simulink model "Quadcopter_Auto_Hinf_Discrete"  (R2016b)
settings: Solver=ode45  StartTime=0.0  StopTime=100  RelTol=1e-3  EnableMultiTasking=on
undefined symbols (not defined in the file): A, B, C, DiscIntNeverNeededParam, g, K_lqi, m, sigbuilder_block, Ts, X0
libraries: simulink x1
settings Model: Creator=Toshiba  LastModifiedBy=AAstudillo
settings DataIOCC: LimitDataPoints=on  SaveFormat=Array  SignalLoggingSaveFormat=ModelDataLogs
settings OptimizationCC: LifeSpan=inf
settings DebuggingCC: SolverPrmCheckMsg=warning  MultiTaskDSMMsg=warning  MultiTaskCondExecSysMsg=none  SFUnexpectedBacktrackingDiag=warning  SFNoUnconditionalDefaultTransitionDiag=warning  SFExecutionAtInitializationDiag=none
settings HardwareCC: ProdBitPerPointer=32  ProdBitPerSizeT=32  ProdBitPerPtrDiffT=32  ProdLargestAtomicFloat=None  ProdIntDivRoundTo=Undefined  ProdEndianess=Unspecified  ProdWordSize=32  ProdHWDeviceType=32-bit Generic
settings ModelReferenceCC: PropagateSignalLabelsOutOfModel=off
settings GRTTargetCC: TargetLangStandard=C89/C90 (ANSI)  GeneratePreprocessorConditionals=Disable all
settings ConfigComp: CovMetricSettings=dw  CovHtmlReporting=on  CovSaveCumulativeToWorkspaceVar=on  CovSaveSingleToWorkspaceVar=on  CovExternalEMLEnable=off

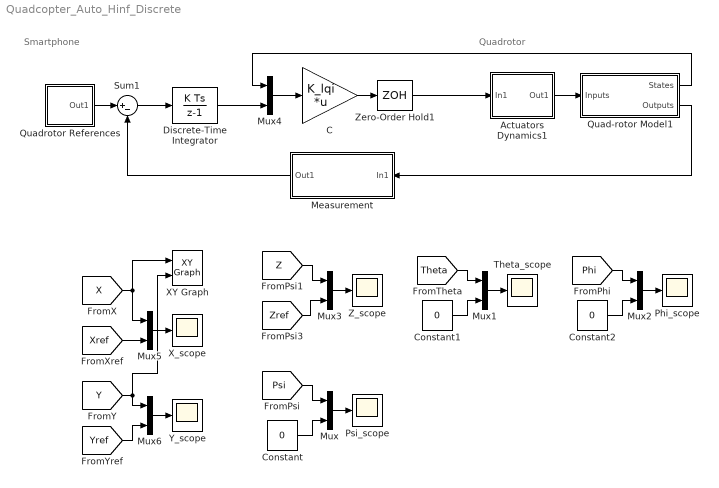
== system Quadcopter_Auto_Hinf_Discrete ==
  note: Quadrotor
  note: Smartphone
  Actuators Dynamics1 : Subsystem
  C : Gain  Gain=K_lqi  Multiplication=Matrix(K*u)
  Constant : Constant  Value=0
  Constant1 : Constant  Value=0
  Constant2 : Constant  Value=0
  Discrete-Time Integrator : DiscreteIntegrator  InitialConditionSetting=State (most efficient)  SampleTime=Ts  UpperSaturationLimit=10  LowerSaturationLimit=-10  ICPrevOutput=DiscIntNeverNeededParam  ICPrevScaledInput=DiscIntNeverNeededParam
  Measurement : Subsystem
  Mux{,1..6} (7 alike) : Mux  Inputs=2
  Phi_scope : Scope
  Psi_scope : Scope
  Quad-rotor Model1 : Subsystem
  Quadrotor References : Subsystem
  Sum1 : Sum  Inputs=|+-
  Theta_scope : Scope
  XY Graph : simulink/Sinks/XY Graph  xmin=-1  xmax=3  ymin=-1  ymax=3  st=Ts
  X_scope : Scope
  Y_scope : Scope
  Z_scope : Scope
  Zero-Order Hold1 : ZeroOrderHold  SampleTime=Ts
  wires:
  Mux/1 -> Psi_scope/1
  Mux1/1 -> Theta_scope/1
  Mux2/1 -> Phi_scope/1
  [Psi] -> Mux/1
  Constant/1 -> Mux/2
  [Theta] -> Mux1/1
  [Phi] -> Mux2/1
  Constant2/1 -> Mux2/2
  Mux3/1 -> Z_scope/1
  [Z] -> Mux3/1
  C/1 -> Zero-Order Hold1/1
  Quad-rotor Model1/1(States) -> Mux4/1
  Mux4/1 -> C/1
  Quadrotor References/1(Out1) -> Sum1/1
  Sum1/1 -> Discrete-Time Integrator/1
  Discrete-Time Integrator/1 -> Mux4/2
  Measurement/1(Out1) -> Sum1/2
  Quad-rotor Model1/2(Outputs) -> Measurement/1(In1)
  Zero-Order Hold1/1 -> Actuators Dynamics1/1(In1)
  Actuators Dynamics1/1(Out1) -> Quad-rotor Model1/1(Inputs)
  Constant1/1 -> Mux1/2
  [Zref] -> Mux3/2
  Mux5/1 -> X_scope/1
  Mux6/1 -> Y_scope/1
  [X] -> XY Graph/1, Mux5/1
  [Xref] -> Mux5/2
  [Y] -> Mux6/1, XY Graph/2
  [Yref] -> Mux6/2

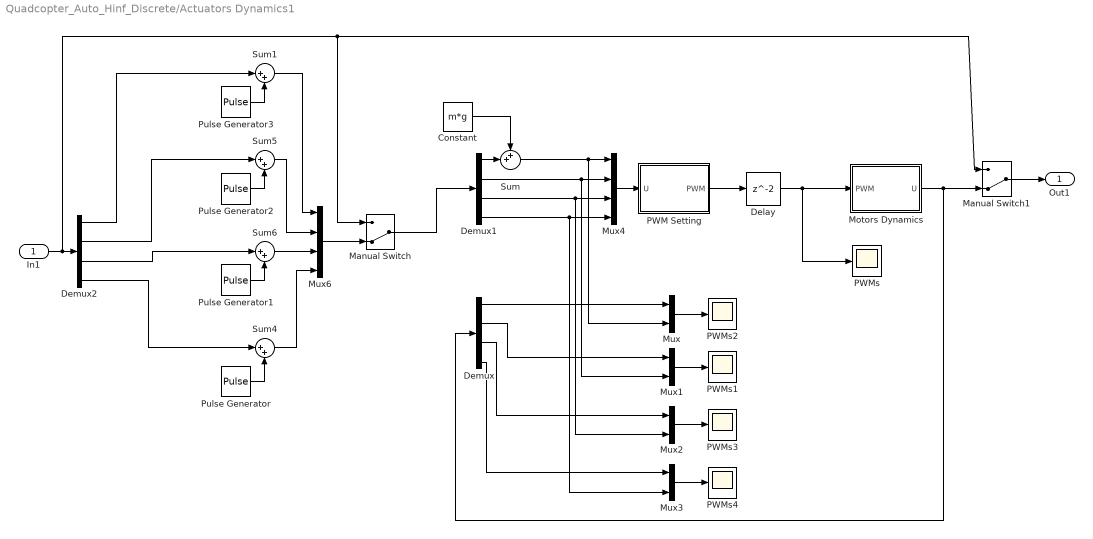
== system Quadcopter_Auto_Hinf_Discrete/Actuators Dynamics1 ==
  In1 : Inport
  Constant : Constant  Value=m*g  VectorParams1D=off  SampleTime=Ts
  Delay : Delay  SampleTime=Ts/10
  Demux : Demux
  Demux1 : Demux
  Demux2 : Demux
  Manual Switch : ManualSwitch  CurrentSetting=0
  Manual Switch1 : ManualSwitch  CurrentSetting=0
  Motors Dynamics : MATLAB Function  TreatAsAtomicUnit=on
  Mux{,1..3} (4 alike) : Mux  Inputs=2
  Mux4 : Mux
  Mux6 : Mux
  PWM Setting : MATLAB Function  TreatAsAtomicUnit=on
  PWMs{,1..4} (5 alike) : Scope
  Pulse Generator : DiscretePulseGenerator  PulseType=Time based  Amplitude=0.05  Period=20  PulseWidth=10  PhaseDelay=10
  Pulse Generator1 : DiscretePulseGenerator  PulseType=Time based  Amplitude=0.1  Period=15  PulseWidth=10  PhaseDelay=5
  Pulse Generator2 : DiscretePulseGenerator  PulseType=Time based  Amplitude=0.2  Period=17  PhaseDelay=15
  Pulse Generator3 : DiscretePulseGenerator  PulseType=Time based  Amplitude=0.1  Period=15  PhaseDelay=15
  Sum : Sum  Inputs=++|
  Sum{1,4..6} (4 alike) : Sum  Inputs=|++
  Out1 : Outport
  wires:
  Motors Dynamics/1(U) -> Manual Switch1/2, Demux/1
  Mux/1 -> PWMs2/1
  Mux1/1 -> PWMs1/1
  Mux2/1 -> PWMs3/1
  Mux3/1 -> PWMs4/1
  Demux/1 -> Mux/1
  Demux/2 -> Mux1/1
  Demux/3 -> Mux2/1
  Demux/4 -> Mux3/1
  Constant/1 -> Sum/1
  Demux1/1 -> Sum/2
  Sum/1 -> Mux/2, Mux4/1
  Demux1/2 -> Mux1/2, Mux4/2
  Demux1/3 -> Mux2/2, Mux4/3
  Demux1/4 -> Mux3/2, Mux4/4
  Mux4/1 -> PWM Setting/1(U)
  PWM Setting/1(PWM) -> Delay/1
  Delay/1 -> PWMs/1, Motors Dynamics/1(PWM)
  Pulse Generator/1 -> Sum4/2
  Pulse Generator1/1 -> Sum6/2
  Pulse Generator2/1 -> Sum5/2
  In1/1 -> Manual Switch1/1, Manual Switch/1, Demux2/1
  Demux2/2 -> Sum5/1
  Demux2/3 -> Sum6/1
  Demux2/4 -> Sum4/1
  Sum5/1 -> Mux6/2
  Sum6/1 -> Mux6/3
  Sum4/1 -> Mux6/4
  Pulse Generator3/1 -> Sum1/2
  Demux2/1 -> Sum1/1
  Sum1/1 -> Mux6/1
  Manual Switch/1 -> Demux1/1
  Mux6/1 -> Manual Switch/2
  Manual Switch1/1 -> Out1/1

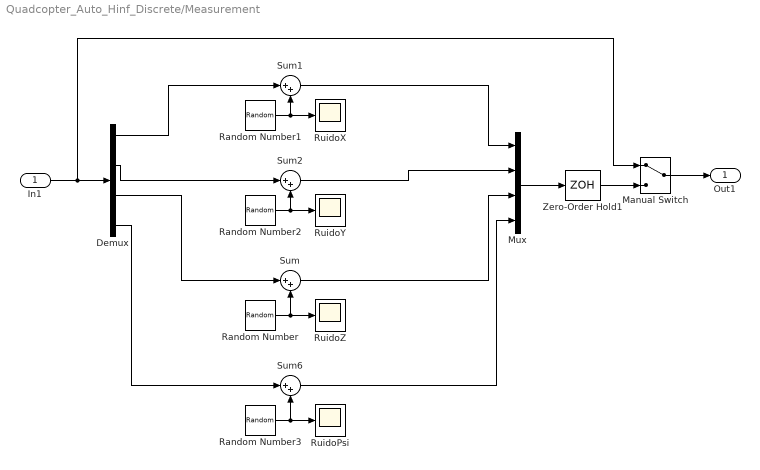
== system Quadcopter_Auto_Hinf_Discrete/Measurement ==
  In1 : Inport
  Demux : Demux
  Manual Switch : ManualSwitch
  Mux : Mux
  Random Number : RandomNumber  Variance=0.005  SampleTime=Ts*100
  Random Number1 : RandomNumber  Variance=0.05  SampleTime=Ts*100
  Random Number2 : RandomNumber  Variance=0.05  SampleTime=Ts*100
  Random Number3 : RandomNumber  Variance=0.00125  SampleTime=Ts
  RuidoPsi : Scope
  RuidoX : Scope
  RuidoY : Scope
  RuidoZ : Scope
  Sum{,1..2,6} (4 alike) : Sum  Inputs=|++
  Zero-Order Hold1 : ZeroOrderHold  SampleTime=Ts
  Out1 : Outport
  wires:
  Mux/1 -> Zero-Order Hold1/1
  Random Number/1 -> Sum/2, RuidoZ/1
  Demux/3 -> Sum/1
  Demux/1 -> Sum1/1
  Random Number2/1 -> RuidoY/1, Sum2/2
  Demux/2 -> Sum2/1
  Random Number1/1 -> RuidoX/1, Sum1/2
  Sum1/1 -> Mux/1
  Sum2/1 -> Mux/2
  Sum/1 -> Mux/3
  Random Number3/1 -> Sum6/2, RuidoPsi/1
  Demux/4 -> Sum6/1
  Sum6/1 -> Mux/4
  Manual Switch/1 -> Out1/1
  Zero-Order Hold1/1 -> Manual Switch/2
  In1/1 -> Manual Switch/1, Demux/1

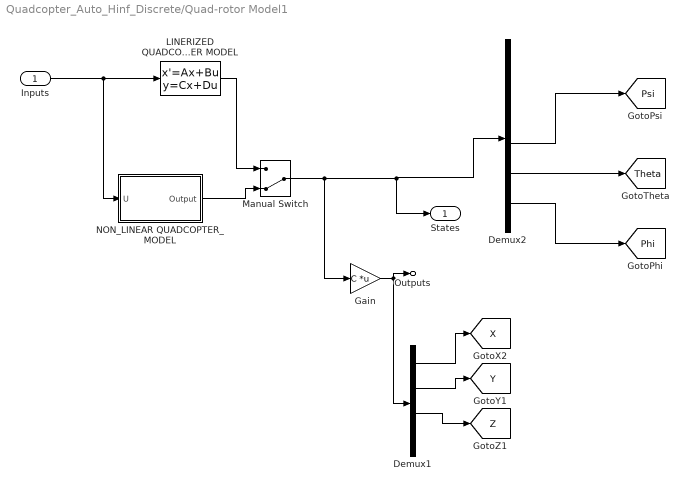
== system Quadcopter_Auto_Hinf_Discrete/Quad-rotor Model1 ==
  Inputs : Inport
  Demux1 : Demux
  Demux2 : Demux  Outputs=12
  Gain : Gain  Gain=C  Multiplication=Matrix(K*u)
  LINERIZED QUADCOPTER MODEL : StateSpace  A=A  B=B  C=eye(12)  D=zeros(12,4)  X0=X0
  Manual Switch : ManualSwitch  CurrentSetting=0
  NON_LINEAR QUADCOPTER_MODEL : Subsystem
  States : Outport
  Outputs : Outport  Port=2
  tag scope: Phi=global, Psi=global, Theta=global, X=global, Y=global, Z=global
  wires:
  Manual Switch/1 -> Gain/1, Demux2/1, States/1
  Gain/1 -> Demux1/1, Outputs/1
  Inputs/1 -> NON_LINEAR QUADCOPTER_MODEL/1(U), LINERIZED QUADCOPTER MODEL/1
  LINERIZED QUADCOPTER MODEL/1 -> Manual Switch/1
  NON_LINEAR QUADCOPTER_MODEL/1("Output ") -> Manual Switch/2
  Demux1/3 -> [Z]
  Demux1/2 -> [Y]
  Demux1/1 -> [X]
  Demux2/7 -> [Psi]
  Demux2/9 -> [Theta]
  Demux2/11 -> [Phi]

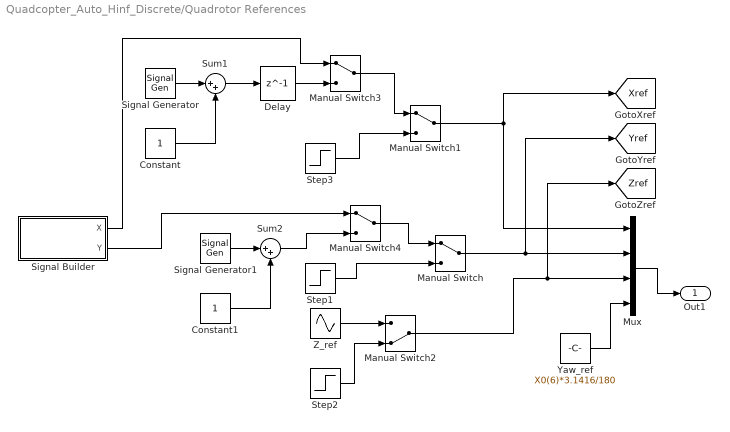
== system Quadcopter_Auto_Hinf_Discrete/Quadrotor References ==
  Constant : Constant
  Constant1 : Constant
  Delay : Delay  DelayLength=1  SampleTime=10
  Manual Switch{,1,3..4} (4 alike) : ManualSwitch
  Manual Switch2 : ManualSwitch  CurrentSetting=0
  Mux : Mux
  Signal Generator : SignalGenerator  WaveForm=square  Amplitude=-1  Frequency=0.025
  Signal Generator1 : SignalGenerator  WaveForm=square  Frequency=0.025
  Signal Builder : Subsystem  Tag=STV Subsys  LoadFcn=sigbuilder_block('load');  StartFcn=sigbuilder_block('start');  StopFcn=sigbuilder_block('stop');  ClipboardFcn=sigbuilder_block('clipboard');  mask(Sigbuilder block){tuvar=[0:10]}
      mask help: Simulink:masks:SigbuilderBlock_MD
      mask init:
      | if ~strcmp(get_param(bdroot(gcbh),'SimulationStatus'),'stopped') tuvar = sigbuilder_block('maskInit'); end
      settings: CopyFcn=sigbuilder_block('copy');  DeleteFcn=sigbuilder_block('delete');  ModelCloseFcn=sigbuilder_block('modelClose');  PreSaveFcn=sigbuilder_block('preSave');  PauseFcn=sigbuilder_block('pause');  ContinueFcn=sigbuilder_block('continue');  NameChangeFcn=sigbuilder_block('namechange');  OpenFcn=sigbuilder_block('open',[6 30 1012.5 447.75 ]);  CloseFcn=sigbuilder_block('close');
      mask Display: plot(0, 0, 100, 100,[2, 2, 32, 32, 2], [68, 8, 8, 68, 68],[32, 2], [38, 38], [32, 19, 2],[53, 60, 44], [32, 17, 17, 2],[16, 16, 31, 31]);txt = getActiveGroup(gcbh);text(2, 100, txt,'verticalAlignment', 'top');
  Step1 : Step  Time=20  Before=1  After=0  SampleTime=0
  Step2 : Step  Time=20  After=0  SampleTime=Ts
  Step3 : Step  Time=20  Before=1  After=0  SampleTime=0
  Sum1 : Sum  Inputs=|++
  Sum2 : Sum  Inputs=|++
  Yaw_ref : Constant  Value=X0(6)*3.1416/180
  Z_ref : Sin  Bias=1  Frequency=3.141592654*0.05  Phase=3.141592654  SampleTime=0
  Out1 : Outport
  tag scope: Xref=global, Yref=global, Zref=global
  wires:
  Mux/1 -> Out1/1
  Yaw_ref/1 -> Mux/4
  Manual Switch1/1 -> Mux/1, [Xref]
  Step3/1 -> Manual Switch1/2
  Step1/1 -> Manual Switch/2
  Manual Switch/1 -> [Yref], Mux/2
  Step2/1 -> Manual Switch2/2
  Z_ref/1 -> Manual Switch2/1
  Manual Switch2/1 -> [Zref], Mux/3
  Signal Generator/1 -> Sum1/1
  Constant/1 -> Sum1/2
  Signal Generator1/1 -> Sum2/1
  Constant1/1 -> Sum2/2
  Sum1/1 -> Delay/1
  Manual Switch3/1 -> Manual Switch1/1
  Delay/1 -> Manual Switch3/2
  Signal Builder/1(X) -> Manual Switch3/1
  Sum2/1 -> Manual Switch4/2
  Manual Switch4/1 -> Manual Switch/1
  Signal Builder/2(Y) -> Manual Switch4/1

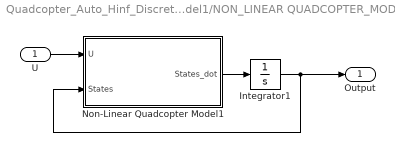
== system Quadcopter_Auto_Hinf_Discrete/Quad-rotor Model1/NON_LINEAR QUADCOPTER_MODEL ==
  U : Inport
  Integrator1 : Integrator  InitialCondition=X0
  Non-Linear Quadcopter Model1 : MATLAB Function  TreatAsAtomicUnit=on
  "Output " : Outport
  wires:
  Non-Linear Quadcopter Model1/1(States_dot) -> Integrator1/1
  Integrator1/1 -> "Output "/1, Non-Linear Quadcopter Model1/2(States)
  U/1 -> Non-Linear Quadcopter Model1/1(U)

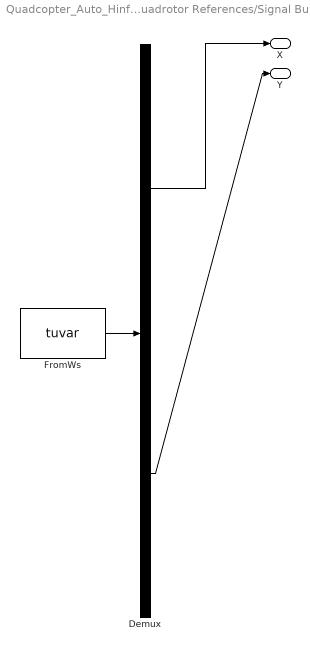
== system Quadcopter_Auto_Hinf_Discrete/Quadrotor References/Signal Builder ==
  Demux : Demux  Tag=STV Demux  Outputs=2
  FromWs : FromWorkspace  Tag=STV FromWs  VariableName=tuvar  SampleTime=0
      SigBuilderData=|
      | common.afterFinalStr = 'Extrapolate'
      | common.sampleTime = 0
      | dataSet.timeRange = [0 135]
      | dataSet.name = 'Group 1'
      | sbobj.Groups.Name = 'Group 1'
      | sbobj.Groups.Signals(1).Name = 'X'
      | sbobj.Groups.Signals(1).XData = [0 10 20 30 40 50 60 70 80 90 100 110 120 135]
      | sbobj.Groups.Signals(1).YData = [0 0 2 2 0 0 2 2 0 0 2 2 0 0]
      | sbobj.Groups.Signals(2).Name = 'Y'
      | sbobj.Groups.Signals(2).XData = [0 20 30 40 50 60 70 80 90 100 110 120 130 135]
      | sbobj.Groups.Signals(2).YData = [0 0 2 2 0 0 2 2 0 0 2 2 0 0]
      | sbobj.Groups.TimeRange = [0 135]
  X : Outport  Tag=STV Outport
  Y : Outport  Tag=STV Outport  Port=2
  wires:
  Demux/1 -> X/1
  FromWs/1 -> Demux/1
  Demux/2 -> Y/1

== matlab function Quadcopter_Auto_Hinf_Discrete/Actuators Dynamics1/PWM Setting ==
  data: U input; PWM output
function PWM = fcn(U)

M_inv = [0.2500  11.9048   -1.4490   -1.4490;
        0.2500  -11.9048   -1.4490    1.4490;
        0.2500   11.9048    1.4490    1.4490;
        0.2500  -11.9048    1.4490   -1.4490];

Force = M_inv*U;

% if Force(1) < 0
%     Force(3) = Force(3) - Force(1);
% end
% if Force(2) < 0
%     Force(4) = Force(4) - Force(2);
% end
% if Force(3) < 0
%     Force(1) = Force(1) - Force(3);
% end
% if Force(4) < 0
%     Force(2) = Force(2) - Force(4);
% end

PWM_1 =  -1.983*(Force(1)^2) + 47.84*Force(1) + 3.835; % PWM [0...255]
PWM_2 =  -1.983*(Force(2)^2) + 47.84*Force(2) + 3.835; % PWM [0...255]
PWM_3 =  -1.983*(Force(3)^2) + 47.84*Force(3) + 3.835; % PWM [0...255]
PWM_4 =  -1.983*(Force(4)^2) + 47.84*Force(4) + 3.835; % PWM [0...255]

if PWM_1 < 0
    PWM_3 = PWM_3 - PWM_1;
end
if PWM_2 < 0
    PWM_4 = PWM_4  - PWM_2;
end
if PWM_3 < 0
    PWM_1 = PWM_1 - PWM_3;
end
if Force(4) < 0
    PWM_2 = PWM_2 - PWM_4 ;
end

PWM_1 = min(255, max(0, PWM_1));
PWM_2 = min(255, max(0, PWM_2));
PWM_3 = min(255, max(0, PWM_3));
PWM_4 = min(255, max(0, PWM_4));

PWM = [PWM_1 PWM_2 PWM_3 PWM_4];

== matlab function Quadcopter_Auto_Hinf_Discrete/Actuators Dynamics1/Motors Dynamics ==
  data: PWM input; U output
function U = fcn(PWM)

F_M1 = (5.441e-5)*(PWM(1)^2) + 0.01586*PWM(1) + 0.014808;
F_M2 = (5.441e-5)*(PWM(2)^2) + 0.01586*PWM(2) + 0.014808;
F_M3 = (5.441e-5)*(PWM(3)^2) + 0.01586*PWM(3) + 0.014808;
F_M4 = (5.441e-5)*(PWM(4)^2) + 0.01586*PWM(4) + 0.014808;

Force = [F_M1 F_M2*1.0256 F_M3 F_M4*1.0256]'; % CCW motors have 2.56 % more efficiency than CW motors

M = [1.0000    1.0000    1.0000    1.0000;
    0.0210   -0.0210    0.0210   -0.0210;
   -0.1725   -0.1725    0.1725    0.1725;
   -0.1725    0.1725    0.1725   -0.1725];


U = M*Force;

== matlab function Quadcopter_Auto_Hinf_Discrete/Quad-rotor Model1/NON_LINEAR QUADCOPTER_MODEL/Non-Linear Quadcopter Model1 ==
  data: U input; States input; States_dot output
function States_dot  = fcn(U, States)

% Gravity constant
              g = 9.807;

              m = 1.568;
              Ixx = 0.0135;
              Iyy = 0.0124;
              Izz = 0.0336;

    %Inputs = U, States
    %Outputs = States_dot  
    %States: X dX Y dY Z dZ Psi dPsi Theta dTheta Phi dPhi
    %        1  2 3  4 5  6  7   8     9      10   11  12
    
    U1 = U(1);
    U2 = U(2);
    U3 = U(3);
    U4 = U(4);

    dX = States(2);
    ddX = (U1/m)*(cos(States(7))*sin(States(9))*cos(States(11)) + sin(States(7))*sin(States(11)));
    %ddX = -States(10)*States(6) + States(8)*States(4) + g*sin(States(9));
    dY = States(4);
    ddY = (U1/m)*(-sin(States(7))*sin(States(9))*cos(States(11)) + cos(States(7))*sin(States(11)));
    %ddY = States(8)*States(2) - States(12)*States(6) + g*cos(States(9))*sin(States(11));
    dZ = States(6);
    ddZ = ((U1/m)*cos(States(9))*cos(States(11))) - g;
    %ddZ = States(10)*States(2) - States(12)*States(4) - g*cos(States(9))*cos(States(11)) + (U1)/m;
    
    dPsi = States(8);
    ddPsi = (((Ixx-Iyy)/Izz)*States(12)*States(10)) + (U2/Izz);
    dTheta = States(10);
    ddTheta = (((Izz-Ixx)/Iyy)*States(12)*States(8)) + (U3/Iyy);
    dPhi = States(12);
    ddPhi = (((Iyy-Izz)/Ixx)*States(10)*States(8)) + (U4/Ixx);

States_dot = [dX, ddX, dY, ddY, dZ, ddZ, dPsi, ddPsi, dTheta, ddTheta, dPhi, ddPhi]';
